simulink model "adcs_v11_log"  (Simulink 7.4)
settings: Solver=ode4  StartTime=0.0  StopTime=80000  FixedStep=s_SIM_STEP_SIZE  RelTol=1e-3
values from neighbouring files (symbols this model uses):
  A = ((T_SIDE + .29)*1e-3)^2    [constants_v13.m]    (also in constants_v15.m; constants_v15_Pow.m; constants_v15_Pow_ss_error.m; constants_v16_integral_kartavya.m)
  Ca_Solar_Drag = 1.4    [constants_v13.m]    (also in constants_v15.m = 0; constants_v15_Pow.m; constants_v15_Pow_ss_error.m; constants_v16_integral_kartavya.m)
  Cd = 2.2    [constants_v13.m]    (also in constants_v15.m = 0; constants_v15_Pow.m; constants_v15_Pow_ss_error.m; constants_v16_integral_kartavya.m)
  check_time = 60000    [constants_v13.m]    (also in constants_v15.m = 10000; constants_v15_Pow_ss_error.m = 10000; constants_v16_integral_kartavya.m = 10000; constants_v16_integral_light_sun_sgp_igrf_power_13Dec2011.m = 10000)
  equinox = datenum('21-Mar-2010 12:0:0')    [constants_v13.m]    (also in constants_v15.m; constants_v15_Pow.m = datenum('20-Mar-2015 12:0:0'); constants_v15_Pow_ss_error.m; constants_v16_integral_kartavya.m)
  err_SGP = 0    [constants_v16_integral_kartavya.m]    (also in constants_v16_integral_light_sun_sgp_igrf_power_13Dec2011.m)
  I_MAX = 0.5    [constants_v13.m]    (also in constants_v15.m; constants_v15_Pow.m; constants_v15_Pow_ss_error.m; constants_v16_integral_kartavya.m)
  I_TORQUER = 3.6 / 7.31    (= 0.492476060192)    [constants_v13.m]    (also in constants_v15.m = 0.272727272727; constants_v15_Pow.m; constants_v15_Pow_ss_error.m; constants_v16_integral_kartavya.m)
  Kd = 2* m_INERTIA / (s_numOrbits * T_ORBIT )    [constants_v13.m]    (also in constants_v15.m = m_INERTIA * (2 + delta)* zeta * w; constants_v15_Pow.m = m_INERTIA * (2 + delta)* zeta * w; constants_v15_Pow_ss_error.m = m_INERTIA * (2 + delta)* zeta * w; constants_v16_integral_kartavya.m = m_INERTIA * (2 + delta)* zeta * w)
  Kdetumb = K_det*eye(3)    [constants_v13.m]    (also in constants_v15.m; constants_v15_Pow.m; constants_v15_Pow_ss_error.m; constants_v16_integral_kartavya.m)
  Kp = m_INERTIA / (s_numOrbits * T_ORBIT * zeta)^2    [constants_v13.m]    (also in constants_v15.m = m_INERTIA * (w*w + 2*delta*zeta^2*w^2); constants_v15_Pow.m = m_INERTIA * (w*w + 2*delta*zeta^2*w^2); constants_v15_Pow_ss_error.m = m_INERTIA * (w*w + 2*delta*zeta^2*w^2); constants_v16_integral_kartavya.m = m_INERTIA * (w*w + 2*delta*zeta^2*w^2))
  m_INERTIA = [Ixx Ixy Ixz; Ixy Iyy Iyz; Ixz Iyz Izz]    [constants_v13.m]    (also in constants_v15.m; constants_v15_Pow.m = 1*[Ixx Ixy Ixz; Ixy Iyy Iyz; Ixz Iyz Izz]; constants_v15_Pow_ss_error.m = 1*[Ixx Ixy Ixz; Ixy Iyy Iyz; Ixz Iyz Izz]; constants_v16_integral_kartavya.m)
  mu = 6.673e-11*5.9742e24    (= 398658366000000)    [constants_v13.m]    (also in constants_v15.m; constants_v15_Pow.m; constants_v15_Pow_ss_error.m; constants_v16_integral_kartavya.m)
  N = 40    [constants_v13.m]    (also in constants_v15.m = 60; constants_v15_Pow.m; constants_v15_Pow_ss_error.m; constants_v16_integral_kartavya.m)
  P_momentum_flux_from_the_sun = 4.4e-6    (= 4.4e-06)    [constants_v13.m]    (also in constants_v15.m = 0; constants_v15_Pow.m; constants_v15_Pow_ss_error.m; constants_v16_integral_kartavya.m)
  q_BI0 = x_fromEnvModel(1:4)'    [OILS_script.m]    (also in OILS_script_OBC_preflight_bounce_back.m; OILS_script_extended.m; OILS_script_preflight_test.m; constants_v13.m = euler2qBI(roll0,pitch0,yaw0))
  s_AU = 159597870610    [constants_v16_integral_kartavya.m]    (also in constants_v16_integral_light_sun_sgp_igrf_power_13Dec2011.m; light_calc.m)
  s_DOY = sime(2)*30 - 30 + sime(3)    [constants_v16_integral_kartavya.m]    (also in constants_v16_integral_light_sun_sgp_igrf_power_13Dec2011.m; precalcs.m = doy(sime(3),sime(2),sime(3)))
  s_FRAME_SIZE = 2    [constants_v13.m]    (also in constants_v15.m; constants_v15_Pow.m; constants_v15_Pow_ss_error.m; constants_v16_integral_kartavya.m)
  s_m_MAX = 0.95    [constants_v13.m]    (also in constants_v15.m; constants_v15_Pow.m; constants_v15_Pow_ss_error.m; constants_v16_integral_kartavya.m)
  s_MAG_B = 2.5e-5    (= 2.5e-05)    [constants_v13.m]    (also in constants_v15.m; constants_v15_Pow.m; constants_v15_Pow_ss_error.m; constants_v16_integral_kartavya.m)
  s_MAGMETER_WEIGHT = .9    (= 0.9)    [constants_v13.m]    (also in constants_v15.m; constants_v15_Pow.m; constants_v15_Pow_ss_error.m; constants_v16_integral_kartavya.m)
  s_Rearth = 6378164    [constants_v16_integral_kartavya.m]    (also in constants_v16_integral_light_sun_sgp_igrf_power_13Dec2011.m; light_calc.m)
  s_Rsun = 695500000    [constants_v16_integral_kartavya.m]    (also in constants_v16_integral_light_sun_sgp_igrf_power_13Dec2011.m; light_calc.m)
  s_SEC = sime(4)*3600 + sime(5)*60 + sime(6)    [constants_v16_integral_kartavya.m]    (also in constants_v16_integral_light_sun_sgp_igrf_power_13Dec2011.m; precalcs.m)
  s_SIM_STEP_SIZE = 0.1    [constants_v13.m]    (also in constants_v15.m; constants_v15_Pow.m; constants_v15_Pow_ss_error.m; constants_v16_integral_kartavya.m)
  s_SS_ADC_gain = 5    [constants_v13.m]    (also in constants_v15.m = 3.3; constants_v15_Pow.m; constants_v15_Pow_ss_error.m; constants_v16_integral_kartavya.m)
  s_SS_ADC_res = 2^12 - 1    (= 4095)    [constants_v13.m]    (also in constants_v15.m = 1023; constants_v15_Pow.m; constants_v15_Pow_ss_error.m; constants_v16_integral_kartavya.m)
  s_SS_MAX_ANGLE = 85    [constants_v13.m]    (also in constants_v15.m = 55; constants_v15_Pow.m; constants_v15_Pow_ss_error.m; constants_v16_integral_kartavya.m)
  s_W_SAT = sqrt(mu/R_e^3)    [constants_v13.m]    (also in constants_v15.m; constants_v15_Pow.m; constants_v15_Pow_ss_error.m; constants_v16_integral_kartavya.m)
  s_x_MAGMETER_BIAS = 50e-9    (= 5e-08)    [constants_v13.m]    (also in constants_v15.m = 0; constants_v15_Pow.m; constants_v15_Pow_ss_error.m; constants_v16_integral_kartavya.m)
  s_YEAR = sime(1) + (sime(2)*30 - 30 + sime(3))/365    [constants_v16_integral_kartavya.m]    (also in constants_v16_integral_light_sun_sgp_igrf_power_13Dec2011.m; precalcs.m = decyear(sime); virtuallabexpt3mag.m = decyear(sime))
  side = 0.26    [constants_v13.m]    (also in constants_v15.m; constants_v15_Pow.m; constants_v15_Pow_ss_error.m; constants_v16_integral_kartavya.m)
  Snum = 6    [constants_v13.m]    (also in constants_v15.m; constants_v15_Pow.m; constants_v15_Pow_ss_error.m; constants_v16_integral_kartavya.m)
  stperut = 1.00273790935    [constants_v16_integral_kartavya.m]    (also in constants_v16_integral_light_sun_sgp_igrf_power_13Dec2011.m; precalcs.m; virtuallabexpt3mag.m)
  t_reset = 600    [constants_v16_integral_kartavya.m]    (also in constants_v16_integral_light_sun_sgp_igrf_power_13Dec2011.m; precalcs.m)
  TLE_epoch = datenum('18-Oct-2015 10:30:0')    [constants_v15.m]    (also in constants_v16_integral_kartavya.m = datenum('18-Oct-2010 10:30:0'); constants_v16_integral_light_sun_sgp_igrf_power_13Dec2011.m = datenum('18-Oct-2010 10:30:0'); precalcs.m)
  today = datenum('18-Oct-2010 10:30:0')    [constants_v13.m]    (also in constants_v15.m; constants_v15_Pow.m = datenum('18-Oct-2015 10:30:0'); constants_v15_Pow_ss_error.m; constants_v16_integral_kartavya.m)
  tol_w = 4e-3    (= 0.004)    [constants_v13.m]    (also in constants_v15.m; constants_v15_Pow.m; constants_v15_Pow_ss_error.m; constants_v16_integral_kartavya.m)
  Ts_display = 6    [constants_v13.m]    (also in constants_v15.m = 2; constants_v15_Pow.m; constants_v15_Pow_ss_error.m; constants_v16_integral_kartavya.m)
  v_COM_to_COP_b = [.2; 1.75; .2]*1e-2    [constants_v13.m]    (also in constants_v15.m = [.2; 1.75; .2]*0e-2; constants_v15_Pow.m; constants_v15_Pow_ss_error.m; constants_v16_integral_kartavya.m)
  v_S1 = [1 0 0]    [constants_v13.m]    (also in constants_v15.m; constants_v15_Pow.m; constants_v15_Pow_ss_error.m; constants_v16_integral_kartavya.m)
  v_S2 = [-1 0 0]    [constants_v13.m]    (also in constants_v15.m; constants_v15_Pow.m; constants_v15_Pow_ss_error.m; constants_v16_integral_kartavya.m)
  v_S3 = [0 1 0]    [constants_v13.m]    (also in constants_v15.m; constants_v15_Pow.m; constants_v15_Pow_ss_error.m; constants_v16_integral_kartavya.m)
  v_S4 = [0 -1 0]    [constants_v13.m]    (also in constants_v15.m; constants_v15_Pow.m; constants_v15_Pow_ss_error.m; constants_v16_integral_kartavya.m)
  v_S5 = [0 0 1]    [constants_v13.m]    (also in constants_v15.m; constants_v15_Pow.m; constants_v15_Pow_ss_error.m; constants_v16_integral_kartavya.m)
  v_S6 = [0 0 -1]    [constants_v13.m]    (also in constants_v15.m; constants_v15_Pow.m; constants_v15_Pow_ss_error.m; constants_v16_integral_kartavya.m)
  v_x_MOUNTING_THETA_ZYX_BODY_TORQUER = [1; 1; 1]* pi/180    [constants_v13.m]    (also in constants_v15.m; constants_v15_Pow.m; constants_v15_Pow_ss_error.m; constants_v16_integral_kartavya.m)
  W_EARTH_ROT = 2*pi/86400    (= 7.27220521664e-05)    [constants_v16_integral_kartavya.m]    (also in constants_v16_integral_light_sun_sgp_igrf_power_13Dec2011.m; precalcs.m; virtuallabexpt3mag.m)
  wx0 = x_fromEnvModel(5)    [OILS_script.m]    (also in OILS_script_OBC_preflight_bounce_back.m; OILS_script_extended.m; OILS_script_preflight_test.m; constants_v13.m = 0.0349065850399)
  wy0 = x_fromEnvModel(6)    [OILS_script.m]    (also in OILS_script_OBC_preflight_bounce_back.m; OILS_script_extended.m; OILS_script_preflight_test.m; constants_v13.m = 0.0174532925199)
  wz0 = x_fromEnvModel(7)    [OILS_script.m]    (also in OILS_script_OBC_preflight_bounce_back.m; OILS_script_extended.m; OILS_script_preflight_test.m; constants_v13.m = -0.0349065850399)
undefined symbols (not defined in the file or in its folder): Earth, s_omega_MAX, s_YEAR_ONLY, tol_pitch, tol_roll, tol_yaw, v_S10, v_S11, v_S12, v_S7, v_S8, v_S9, v_Si0, WGS84
libraries: commnoisgen2 x15, aerolibutil x7, aerolibtransform2 x5, dspsigops x5, powerlib_extras x3, aerolibgravity2 x2, aerolibatmos2 x1, dspmtrx3 x1, simulink x1
(part 2 of 3)

== system adcs_v11_log/Satellite Computations I Propagators/WMM/Subsystem ==
  Clock : Clock
      settings: Decimation=10
  m_DCM_ECI-ECEF2 : Stateflow chart
  today : Constant  Value=today  OutDataType=sfix(16)  OutScaling=2^0
  today1 : Constant  Value=equinox  OutDataType=sfix(16)  OutScaling=2^0
  today2 : Constant  Value=stperut  OutDataType=sfix(16)  OutScaling=2^0
  today3 : Constant  Value=W_EARTH_ROT  OutDataType=sfix(16)  OutScaling=2^0
  TEI : Outport
  wires:
  m_DCM_ECI-ECEF2/1(TEI) -> TEI/1
  Clock/1 -> m_DCM_ECI-ECEF2/5(t)
  today3/1 -> m_DCM_ECI-ECEF2/4(W_EARTH_ROT)
  today2/1 -> m_DCM_ECI-ECEF2/3(stperut)
  today1/1 -> m_DCM_ECI-ECEF2/2(equinox)
  today/1 -> m_DCM_ECI-ECEF2/1(today)

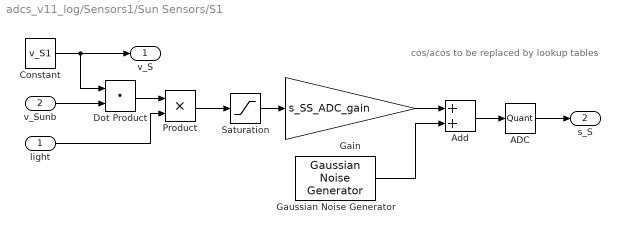
== system adcs_v11_log/Sensors1/Sun Sensors/S1 ==
  note: cos/acos to be replaced by lookup tables
  light : Inport  OutDataType=sfix(16)  OutScaling=2^0
  v_Sunb : Inport  Port=2  OutDataType=sfix(16)  OutScaling=2^0
  ADC : Quantizer  QuantizationInterval=1/s_SS_ADC_res
  Add : Sum  OutDataType=sfix(16)  OutScaling=2^-10
  Constant : Constant  Value=v_S1  OutDataType=sfix(16)  OutScaling=2^0
  Dot Product : DotProduct  OutDataType=sfix(16)  OutScaling=2^-10  InputSameDT=on  OutDataTypeStr=Inherit: Inherit via internal rule
  Gain : Gain  Gain=s_SS_ADC_gain  ParameterDataType=sfix(16)  ParameterScaling=2^0  OutDataType=sfix(16)  OutScaling=2^0
  Gaussian Noise Generator : commnoisgen2/Gaussian Noise Generator  SystemSampleTime=-1  m=0  d=s_x_SUNSENSOR  s=41  Ts=s_SIM_STEP_SIZE  frameBased=off  sampPerFrame=1  orient=off  outDataType=double
  Product : Product  OutDataType=fixdt(1, 16)  OutScaling=2^0  RndMeth=Zero
  Saturation : Saturate  UpperLimit=inf  LowerLimit=0  OutDataType=sfix(16)  OutScaling=2^0
  v_S : Outport  OutDataType=sfix(16)  OutScaling=2^0
  s_S : Outport  Port=2  OutDataType=sfix(16)  OutScaling=2^0
  wires:
  light/1 -> Product/2
  Product/1 -> Saturation/1
  Dot Product/1 -> Product/1
  v_Sunb/1 -> Dot Product/2
  Saturation/1 -> Gain/1
  Constant/1 -> v_S/1, Dot Product/1
  Gaussian Noise Generator/1 -> Add/2
  Gain/1 -> Add/1
  Add/1 -> ADC/1
  ADC/1 -> s_S/1

== system adcs_v11_log/Sensors1/Sun Sensors/S10 ==
  note: cos/acos to be replaced by lookup tables
  light : Inport  OutDataType=sfix(16)  OutScaling=2^0
  v_Sunb : Inport  Port=2  OutDataType=sfix(16)  OutScaling=2^0
  ADC : Quantizer  QuantizationInterval=1/s_SS_ADC_res
  Add : Sum  OutDataType=sfix(16)  OutScaling=2^-10
  Constant : Constant  Value=v_S10  OutDataType=sfix(16)  OutScaling=2^0
  Dot Product : DotProduct  OutDataType=sfix(16)  OutScaling=2^-10  InputSameDT=on  OutDataTypeStr=Inherit: Inherit via internal rule
  Gain : Gain  Gain=s_SS_ADC_gain  ParameterDataType=sfix(16)  ParameterScaling=2^0  OutDataType=sfix(16)  OutScaling=2^0
  Gaussian Noise Generator : commnoisgen2/Gaussian Noise Generator  SystemSampleTime=-1  m=0  d=s_x_SUNSENSOR  s=41  Ts=s_SIM_STEP_SIZE  frameBased=off  sampPerFrame=1  orient=off  outDataType=double
  Product : Product  OutDataType=fixdt(1, 16)  OutScaling=2^0  RndMeth=Zero
  Saturation : Saturate  UpperLimit=inf  LowerLimit=0  OutDataType=sfix(16)  OutScaling=2^0
  v_S : Outport  OutDataType=sfix(16)  OutScaling=2^0
  s_S : Outport  Port=2  OutDataType=sfix(16)  OutScaling=2^0
  wires:
  ADC/1 -> s_S/1
  Add/1 -> ADC/1
  Gain/1 -> Add/1
  Gaussian Noise Generator/1 -> Add/2
  Constant/1 -> Dot Product/1, v_S/1
  Saturation/1 -> Gain/1
  v_Sunb/1 -> Dot Product/2
  Dot Product/1 -> Product/1
  Product/1 -> Saturation/1
  light/1 -> Product/2

== system adcs_v11_log/Sensors1/Sun Sensors/S11 ==
  note: cos/acos to be replaced by lookup tables
  light : Inport  OutDataType=sfix(16)  OutScaling=2^0
  v_Sunb : Inport  Port=2  OutDataType=sfix(16)  OutScaling=2^0
  ADC : Quantizer  QuantizationInterval=1/s_SS_ADC_res
  Add : Sum  OutDataType=sfix(16)  OutScaling=2^-10
  Constant : Constant  Value=v_S11  OutDataType=sfix(16)  OutScaling=2^0
  Dot Product : DotProduct  OutDataType=sfix(16)  OutScaling=2^-10  InputSameDT=on  OutDataTypeStr=Inherit: Inherit via internal rule
  Gain : Gain  Gain=s_SS_ADC_gain  ParameterDataType=sfix(16)  ParameterScaling=2^0  OutDataType=sfix(16)  OutScaling=2^0
  Gaussian Noise Generator : commnoisgen2/Gaussian Noise Generator  SystemSampleTime=-1  m=0  d=s_x_SUNSENSOR  s=41  Ts=s_SIM_STEP_SIZE  frameBased=off  sampPerFrame=1  orient=off  outDataType=double
  Product : Product  OutDataType=fixdt(1, 16)  OutScaling=2^0  RndMeth=Zero
  Saturation : Saturate  UpperLimit=inf  LowerLimit=0  OutDataType=sfix(16)  OutScaling=2^0
  v_S : Outport  OutDataType=sfix(16)  OutScaling=2^0
  s_S : Outport  Port=2  OutDataType=sfix(16)  OutScaling=2^0
  wires:
  light/1 -> Product/2
  Product/1 -> Saturation/1
  Dot Product/1 -> Product/1
  v_Sunb/1 -> Dot Product/2
  Saturation/1 -> Gain/1
  Constant/1 -> v_S/1, Dot Product/1
  Gaussian Noise Generator/1 -> Add/2
  Gain/1 -> Add/1
  Add/1 -> ADC/1
  ADC/1 -> s_S/1

== system adcs_v11_log/Sensors1/Sun Sensors/S12 ==
  note: cos/acos to be replaced by lookup tables
  light : Inport  OutDataType=sfix(16)  OutScaling=2^0
  v_Sunb : Inport  Port=2  OutDataType=sfix(16)  OutScaling=2^0
  ADC : Quantizer  QuantizationInterval=1/s_SS_ADC_res
  Add : Sum  OutDataType=sfix(16)  OutScaling=2^-10
  Constant : Constant  Value=v_S12  OutDataType=sfix(16)  OutScaling=2^0
  Dot Product : DotProduct  OutDataType=sfix(16)  OutScaling=2^-10  InputSameDT=on  OutDataTypeStr=Inherit: Inherit via internal rule
  Gain : Gain  Gain=s_SS_ADC_gain  ParameterDataType=sfix(16)  ParameterScaling=2^0  OutDataType=sfix(16)  OutScaling=2^0
  Gaussian Noise Generator : commnoisgen2/Gaussian Noise Generator  SystemSampleTime=-1  m=0  d=s_x_SUNSENSOR  s=41  Ts=s_SIM_STEP_SIZE  frameBased=off  sampPerFrame=1  orient=off  outDataType=double
  Product : Product  OutDataType=fixdt(1, 16)  OutScaling=2^0  RndMeth=Zero
  Saturation : Saturate  UpperLimit=inf  LowerLimit=0  OutDataType=sfix(16)  OutScaling=2^0
  v_S : Outport  OutDataType=sfix(16)  OutScaling=2^0
  s_S : Outport  Port=2  OutDataType=sfix(16)  OutScaling=2^0
  wires:
  ADC/1 -> s_S/1
  Add/1 -> ADC/1
  Gain/1 -> Add/1
  Gaussian Noise Generator/1 -> Add/2
  Constant/1 -> Dot Product/1, v_S/1
  Saturation/1 -> Gain/1
  v_Sunb/1 -> Dot Product/2
  Dot Product/1 -> Product/1
  Product/1 -> Saturation/1
  light/1 -> Product/2

== system adcs_v11_log/Sensors1/Sun Sensors/S2 ==
  note: cos/acos to be replaced by lookup tables
  light : Inport  OutDataType=sfix(16)  OutScaling=2^0
  v_Sunb : Inport  Port=2  OutDataType=sfix(16)  OutScaling=2^0
  ADC : Quantizer  QuantizationInterval=1/s_SS_ADC_res
  Add : Sum  OutDataType=sfix(16)  OutScaling=2^-10
  Constant : Constant  Value=v_S2  OutDataType=sfix(16)  OutScaling=2^0
  Dot Product : DotProduct  OutDataType=sfix(16)  OutScaling=2^-10  InputSameDT=on  OutDataTypeStr=Inherit: Inherit via internal rule
  Gain : Gain  Gain=s_SS_ADC_gain  ParameterDataType=sfix(16)  ParameterScaling=2^0  OutDataType=sfix(16)  OutScaling=2^0
  Gaussian Noise Generator : commnoisgen2/Gaussian Noise Generator  SystemSampleTime=-1  m=0  d=s_x_SUNSENSOR  s=41  Ts=s_SIM_STEP_SIZE  frameBased=off  sampPerFrame=1  orient=off  outDataType=double
  Product : Product  OutDataType=fixdt(1, 16)  OutScaling=2^0  RndMeth=Zero
  Saturation : Saturate  UpperLimit=inf  LowerLimit=0  OutDataType=sfix(16)  OutScaling=2^0
  v_S : Outport  OutDataType=sfix(16)  OutScaling=2^0
  s_S : Outport  Port=2  OutDataType=sfix(16)  OutScaling=2^0
  wires:
  ADC/1 -> s_S/1
  Add/1 -> ADC/1
  Gain/1 -> Add/1
  Gaussian Noise Generator/1 -> Add/2
  Constant/1 -> Dot Product/1, v_S/1
  Saturation/1 -> Gain/1
  v_Sunb/1 -> Dot Product/2
  Dot Product/1 -> Product/1
  Product/1 -> Saturation/1
  light/1 -> Product/2

== system adcs_v11_log/Sensors1/Sun Sensors/S3 ==
  note: cos/acos to be replaced by lookup tables
  light : Inport  OutDataType=sfix(16)  OutScaling=2^0
  v_Sunb : Inport  Port=2  OutDataType=sfix(16)  OutScaling=2^0
  ADC : Quantizer  QuantizationInterval=1/s_SS_ADC_res
  Add : Sum  OutDataType=sfix(16)  OutScaling=2^-10
  Constant : Constant  Value=v_S3  OutDataType=sfix(16)  OutScaling=2^0
  Dot Product : DotProduct  OutDataType=sfix(16)  OutScaling=2^-10  InputSameDT=on  OutDataTypeStr=Inherit: Inherit via internal rule
  Gain : Gain  Gain=s_SS_ADC_gain  ParameterDataType=sfix(16)  ParameterScaling=2^0  OutDataType=sfix(16)  OutScaling=2^0
  Gaussian Noise Generator : commnoisgen2/Gaussian Noise Generator  SystemSampleTime=-1  m=0  d=s_x_SUNSENSOR  s=41  Ts=s_SIM_STEP_SIZE  frameBased=off  sampPerFrame=1  orient=off  outDataType=double
  Product : Product  OutDataType=fixdt(1, 16)  OutScaling=2^0  RndMeth=Zero
  Saturation : Saturate  UpperLimit=inf  LowerLimit=0  OutDataType=sfix(16)  OutScaling=2^0
  v_S : Outport  OutDataType=sfix(16)  OutScaling=2^0
  s_S : Outport  Port=2  OutDataType=sfix(16)  OutScaling=2^0
  wires:
  light/1 -> Product/2
  Product/1 -> Saturation/1
  Dot Product/1 -> Product/1
  v_Sunb/1 -> Dot Product/2
  Saturation/1 -> Gain/1
  Constant/1 -> v_S/1, Dot Product/1
  Gaussian Noise Generator/1 -> Add/2
  Gain/1 -> Add/1
  Add/1 -> ADC/1
  ADC/1 -> s_S/1

== system adcs_v11_log/Sensors1/Sun Sensors/S4 ==
  note: cos/acos to be replaced by lookup tables
  light : Inport  OutDataType=sfix(16)  OutScaling=2^0
  v_Sunb : Inport  Port=2  OutDataType=sfix(16)  OutScaling=2^0
  ADC : Quantizer  QuantizationInterval=1/s_SS_ADC_res
  Add : Sum  OutDataType=sfix(16)  OutScaling=2^-10
  Constant : Constant  Value=v_S4  OutDataType=sfix(16)  OutScaling=2^0
  Dot Product : DotProduct  OutDataType=sfix(16)  OutScaling=2^-10  InputSameDT=on  OutDataTypeStr=Inherit: Inherit via internal rule
  Gain : Gain  Gain=s_SS_ADC_gain  ParameterDataType=sfix(16)  ParameterScaling=2^0  OutDataType=sfix(16)  OutScaling=2^0
  Gaussian Noise Generator : commnoisgen2/Gaussian Noise Generator  SystemSampleTime=-1  m=0  d=s_x_SUNSENSOR  s=41  Ts=s_SIM_STEP_SIZE  frameBased=off  sampPerFrame=1  orient=off  outDataType=double
  Product : Product  OutDataType=fixdt(1, 16)  OutScaling=2^0  RndMeth=Zero
  Saturation : Saturate  UpperLimit=inf  LowerLimit=0  OutDataType=sfix(16)  OutScaling=2^0
  v_S : Outport  OutDataType=sfix(16)  OutScaling=2^0
  s_S : Outport  Port=2  OutDataType=sfix(16)  OutScaling=2^0
  wires:
  ADC/1 -> s_S/1
  Add/1 -> ADC/1
  Gain/1 -> Add/1
  Gaussian Noise Generator/1 -> Add/2
  Constant/1 -> Dot Product/1, v_S/1
  Saturation/1 -> Gain/1
  v_Sunb/1 -> Dot Product/2
  Dot Product/1 -> Product/1
  Product/1 -> Saturation/1
  light/1 -> Product/2

== system adcs_v11_log/Sensors1/Sun Sensors/S5 ==
  note: cos/acos to be replaced by lookup tables
  light : Inport  OutDataType=sfix(16)  OutScaling=2^0
  v_Sunb : Inport  Port=2  OutDataType=sfix(16)  OutScaling=2^0
  ADC : Quantizer  QuantizationInterval=1/s_SS_ADC_res
  Add : Sum  OutDataType=sfix(16)  OutScaling=2^-10
  Constant : Constant  Value=v_S5  OutDataType=sfix(16)  OutScaling=2^0
  Dot Product : DotProduct  OutDataType=sfix(16)  OutScaling=2^-10  InputSameDT=on  OutDataTypeStr=Inherit: Inherit via internal rule
  Gain : Gain  Gain=s_SS_ADC_gain  ParameterDataType=sfix(16)  ParameterScaling=2^0  OutDataType=sfix(16)  OutScaling=2^0
  Gaussian Noise Generator : commnoisgen2/Gaussian Noise Generator  SystemSampleTime=-1  m=0  d=s_x_SUNSENSOR  s=41  Ts=s_SIM_STEP_SIZE  frameBased=off  sampPerFrame=1  orient=off  outDataType=double
  Product : Product  OutDataType=fixdt(1, 16)  OutScaling=2^0  RndMeth=Zero
  Saturation : Saturate  UpperLimit=inf  LowerLimit=0  OutDataType=sfix(16)  OutScaling=2^0
  v_S : Outport  OutDataType=sfix(16)  OutScaling=2^0
  s_S : Outport  Port=2  OutDataType=sfix(16)  OutScaling=2^0
  wires:
  light/1 -> Product/2
  Product/1 -> Saturation/1
  Dot Product/1 -> Product/1
  v_Sunb/1 -> Dot Product/2
  Saturation/1 -> Gain/1
  Constant/1 -> v_S/1, Dot Product/1
  Gaussian Noise Generator/1 -> Add/2
  Gain/1 -> Add/1
  Add/1 -> ADC/1
  ADC/1 -> s_S/1

== system adcs_v11_log/Sensors1/Sun Sensors/S6 ==
  note: cos/acos to be replaced by lookup tables
  light : Inport  OutDataType=sfix(16)  OutScaling=2^0
  v_Sunb : Inport  Port=2  OutDataType=sfix(16)  OutScaling=2^0
  ADC : Quantizer  QuantizationInterval=1/s_SS_ADC_res
  Add : Sum  OutDataType=sfix(16)  OutScaling=2^-10
  Constant : Constant  Value=v_S6  OutDataType=sfix(16)  OutScaling=2^0
  Dot Product : DotProduct  OutDataType=sfix(16)  OutScaling=2^-10  InputSameDT=on  OutDataTypeStr=Inherit: Inherit via internal rule
  Gain : Gain  Gain=s_SS_ADC_gain  ParameterDataType=sfix(16)  ParameterScaling=2^0  OutDataType=sfix(16)  OutScaling=2^0
  Gaussian Noise Generator : commnoisgen2/Gaussian Noise Generator  SystemSampleTime=-1  m=0  d=s_x_SUNSENSOR  s=41  Ts=s_SIM_STEP_SIZE  frameBased=off  sampPerFrame=1  orient=off  outDataType=double
  Product : Product  OutDataType=fixdt(1, 16)  OutScaling=2^0  RndMeth=Zero
  Saturation : Saturate  UpperLimit=inf  LowerLimit=0  OutDataType=sfix(16)  OutScaling=2^0
  v_S : Outport  OutDataType=sfix(16)  OutScaling=2^0
  s_S : Outport  Port=2  OutDataType=sfix(16)  OutScaling=2^0
  wires:
  ADC/1 -> s_S/1
  Add/1 -> ADC/1
  Gain/1 -> Add/1
  Gaussian Noise Generator/1 -> Add/2
  Constant/1 -> Dot Product/1, v_S/1
  Saturation/1 -> Gain/1
  v_Sunb/1 -> Dot Product/2
  Dot Product/1 -> Product/1
  Product/1 -> Saturation/1
  light/1 -> Product/2

== system adcs_v11_log/Sensors1/Sun Sensors/S7 ==
  note: cos/acos to be replaced by lookup tables
  light : Inport  OutDataType=sfix(16)  OutScaling=2^0
  v_Sunb : Inport  Port=2  OutDataType=sfix(16)  OutScaling=2^0
  ADC : Quantizer  QuantizationInterval=1/s_SS_ADC_res
  Add : Sum  OutDataType=sfix(16)  OutScaling=2^-10
  Constant : Constant  Value=v_S7  OutDataType=sfix(16)  OutScaling=2^0
  Dot Product : DotProduct  OutDataType=sfix(16)  OutScaling=2^-10  InputSameDT=on  OutDataTypeStr=Inherit: Inherit via internal rule
  Gain : Gain  Gain=s_SS_ADC_gain  ParameterDataType=sfix(16)  ParameterScaling=2^0  OutDataType=sfix(16)  OutScaling=2^0
  Gaussian Noise Generator : commnoisgen2/Gaussian Noise Generator  SystemSampleTime=-1  m=0  d=s_x_SUNSENSOR  s=41  Ts=s_SIM_STEP_SIZE  frameBased=off  sampPerFrame=1  orient=off  outDataType=double
  Product : Product  OutDataType=fixdt(1, 16)  OutScaling=2^0  RndMeth=Zero
  Saturation : Saturate  UpperLimit=inf  LowerLimit=0  OutDataType=sfix(16)  OutScaling=2^0
  v_S : Outport  OutDataType=sfix(16)  OutScaling=2^0
  s_S : Outport  Port=2  OutDataType=sfix(16)  OutScaling=2^0
  wires:
  light/1 -> Product/2
  Product/1 -> Saturation/1
  Dot Product/1 -> Product/1
  v_Sunb/1 -> Dot Product/2
  Saturation/1 -> Gain/1
  Constant/1 -> v_S/1, Dot Product/1
  Gaussian Noise Generator/1 -> Add/2
  Gain/1 -> Add/1
  Add/1 -> ADC/1
  ADC/1 -> s_S/1

== system adcs_v11_log/Sensors1/Sun Sensors/S8 ==
  note: cos/acos to be replaced by lookup tables
  light : Inport  OutDataType=sfix(16)  OutScaling=2^0
  v_Sunb : Inport  Port=2  OutDataType=sfix(16)  OutScaling=2^0
  ADC : Quantizer  QuantizationInterval=1/s_SS_ADC_res
  Add : Sum  OutDataType=sfix(16)  OutScaling=2^-10
  Constant : Constant  Value=v_S8  OutDataType=sfix(16)  OutScaling=2^0
  Dot Product : DotProduct  OutDataType=sfix(16)  OutScaling=2^-10  InputSameDT=on  OutDataTypeStr=Inherit: Inherit via internal rule
  Gain : Gain  Gain=s_SS_ADC_gain  ParameterDataType=sfix(16)  ParameterScaling=2^0  OutDataType=sfix(16)  OutScaling=2^0
  Gaussian Noise Generator : commnoisgen2/Gaussian Noise Generator  SystemSampleTime=-1  m=0  d=s_x_SUNSENSOR  s=41  Ts=s_SIM_STEP_SIZE  frameBased=off  sampPerFrame=1  orient=off  outDataType=double
  Product : Product  OutDataType=fixdt(1, 16)  OutScaling=2^0  RndMeth=Zero
  Saturation : Saturate  UpperLimit=inf  LowerLimit=0  OutDataType=sfix(16)  OutScaling=2^0
  v_S : Outport  OutDataType=sfix(16)  OutScaling=2^0
  s_S : Outport  Port=2  OutDataType=sfix(16)  OutScaling=2^0
  wires:
  ADC/1 -> s_S/1
  Add/1 -> ADC/1
  Gain/1 -> Add/1
  Gaussian Noise Generator/1 -> Add/2
  Constant/1 -> Dot Product/1, v_S/1
  Saturation/1 -> Gain/1
  v_Sunb/1 -> Dot Product/2
  Dot Product/1 -> Product/1
  Product/1 -> Saturation/1
  light/1 -> Product/2

== system adcs_v11_log/Sensors1/Sun Sensors/S9 ==
  note: cos/acos to be replaced by lookup tables
  light : Inport  OutDataType=sfix(16)  OutScaling=2^0
  v_Sunb : Inport  Port=2  OutDataType=sfix(16)  OutScaling=2^0
  ADC : Quantizer  QuantizationInterval=1/s_SS_ADC_res
  Add : Sum  OutDataType=sfix(16)  OutScaling=2^-10
  Constant : Constant  Value=v_S9  OutDataType=sfix(16)  OutScaling=2^0
  Dot Product : DotProduct  OutDataType=sfix(16)  OutScaling=2^-10  InputSameDT=on  OutDataTypeStr=Inherit: Inherit via internal rule
  Gain : Gain  Gain=s_SS_ADC_gain  ParameterDataType=sfix(16)  ParameterScaling=2^0  OutDataType=sfix(16)  OutScaling=2^0
  Gaussian Noise Generator : commnoisgen2/Gaussian Noise Generator  SystemSampleTime=-1  m=0  d=s_x_SUNSENSOR  s=41  Ts=s_SIM_STEP_SIZE  frameBased=off  sampPerFrame=1  orient=off  outDataType=double
  Product : Product  OutDataType=fixdt(1, 16)  OutScaling=2^0  RndMeth=Zero
  Saturation : Saturate  UpperLimit=inf  LowerLimit=0  OutDataType=sfix(16)  OutScaling=2^0
  v_S : Outport  OutDataType=sfix(16)  OutScaling=2^0
  s_S : Outport  Port=2  OutDataType=sfix(16)  OutScaling=2^0
  wires:
  light/1 -> Product/2
  Product/1 -> Saturation/1
  Dot Product/1 -> Product/1
  v_Sunb/1 -> Dot Product/2
  Saturation/1 -> Gain/1
  Constant/1 -> v_S/1, Dot Product/1
  Gaussian Noise Generator/1 -> Add/2
  Gain/1 -> Add/1
  Add/1 -> ADC/1
  ADC/1 -> s_S/1

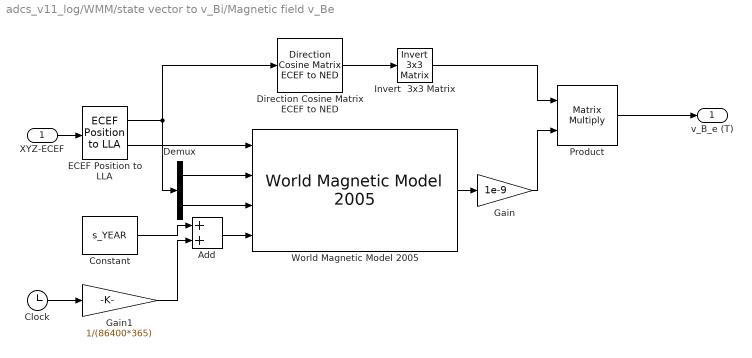
== system adcs_v11_log/WMM/state vector to v_Bi/Magnetic field v_Be ==
  XYZ-ECEF : Inport  OutDataType=sfix(16)  OutScaling=2^0
  Add : Sum  OutDataType=sfix(16)  OutScaling=2^-10
  Clock : Clock
      settings: Decimation=10
  Constant : Constant  Value=s_YEAR  OutDataType=sfix(16)  OutScaling=2^0
  Demux : Demux  Outputs=2
  Direction Cosine Matrix ECEF to NED : aerolibtransform2/Direction Cosine Matrix ECEF to NED  SystemSampleTime=-1
  ECEF Position to LLA : aerolibtransform2/ECEF Position to LLA  SystemSampleTime=-1  units=Metric (MKS)  ptype=Earth (WGS84)  F=1/298.257223563  R=6378137
  Gain : Gain  Gain=1e-9  ParameterDataType=sfix(16)  ParameterScaling=2^0  OutDataType=sfix(16)  OutScaling=2^0
  Gain1 : Gain  Gain=1/(86400*365)  ParameterDataType=sfix(16)  ParameterScaling=2^0  OutDataType=sfix(16)  OutScaling=2^0
  Invert  3x3 Matrix : aerolibutil/Invert  3x3 Matrix  SystemSampleTime=-1
  Product : Product  Multiplication=Matrix(*)  OutDataType=sfix(16)  OutScaling=2^0  RndMeth=Zero
  World Magnetic Model 2005 : aerolibgravity2/World Magnetic Model 2005  SystemSampleTime=-1  units=Metric (MKS)  time_in=on  month=January  day=1  year=2005  action=Error  h_out=off  dec_out=off  inc_out=off  ti_out=off
  "v_B_e (T) " : Outport  OutDataType=sfix(16)  OutScaling=2^0
  wires:
  Gain1/1 -> Add/2
  Clock/1 -> Gain1/1
  Add/1 -> World Magnetic Model 2005/4
  Constant/1 -> Add/1
  XYZ-ECEF/1 -> ECEF Position to LLA/1
  ECEF Position to LLA/1 -> Demux/1, Direction Cosine Matrix ECEF to NED/1
  ECEF Position to LLA/2 -> World Magnetic Model 2005/1
  Demux/1 -> World Magnetic Model 2005/2
  Demux/2 -> World Magnetic Model 2005/3
  Direction Cosine Matrix ECEF to NED/1 -> Invert  3x3 Matrix/1
  Invert  3x3 Matrix/1 -> Product/1
  Product/1 -> "v_B_e (T) "/1
  World Magnetic Model 2005/1 -> Gain/1
  Gain/1 -> Product/2

== system adcs_v11_log/WMM/state vector to v_Bi/Subsystem ==
  Clock : Clock
      settings: Decimation=10
  m_DCM_ECI-ECEF2 : Stateflow chart
  today : Constant  Value=today  OutDataType=sfix(16)  OutScaling=2^0
  today1 : Constant  Value=equinox  OutDataType=sfix(16)  OutScaling=2^0
  today2 : Constant  Value=stperut  OutDataType=sfix(16)  OutScaling=2^0
  today3 : Constant  Value=W_EARTH_ROT  OutDataType=sfix(16)  OutScaling=2^0
  TEI : Outport
  wires:
  m_DCM_ECI-ECEF2/1(TEI) -> TEI/1
  Clock/1 -> m_DCM_ECI-ECEF2/5(t)
  today3/1 -> m_DCM_ECI-ECEF2/4(W_EARTH_ROT)
  today2/1 -> m_DCM_ECI-ECEF2/3(stperut)
  today1/1 -> m_DCM_ECI-ECEF2/2(equinox)
  today/1 -> m_DCM_ECI-ECEF2/1(today)

== matlab function Torquer/Embedded MATLAB Function4 ==
  data: euler input double; DCM output double
function DCM  = f(euler)
% This block supports the Embedded MATLAB subset.
% See the help menu for details. 

roll = euler(1);
pitch = euler(2);
yaw = euler(3);

rot_x = [  1         0           0;...
             0         cos(roll)  sin(roll);...
             0        -sin(roll)  cos(roll)];
         
rot_y = [cos(pitch)   0       -sin(pitch);...
            0           1        0;...
           sin(pitch)   0        cos(pitch)];
       
rot_z = [ cos(yaw) sin(yaw) 0;...
           -sin(yaw) cos(yaw) 0;...
            0        0            1];
         
DCM  = rot_z *  rot_y *  rot_x;

== matlab function Embedded MATLAB Function ==
  data: x input double; u input double; xdot output double; m_INERTIA parameter double
function xdot = fcn(x, u, m_INERTIA)
% This block supports the Embedded MATLAB subset.
% See the help menu for details. 

q = x(1:4);
w = x(5:7);

W = ...
    [ 0 w(3) -w(2) w(1);
      -w(3) 0 w(1) w(2);
      w(2) -w(1) 0 w(3);
      -w(1) -w(2) -w(3) 0];
  
  qdot = 0.5 * W * q;
  wdot = inv(m_INERTIA)*( u - cross( w, m_INERTIA*w ) );
  
  xdot = [qdot; wdot];

== matlab function Subsystem/Sun Vector Propagator ==
  data: today input double; v_Sun_i output double; t input double
function v_Sun_i = fcn(today,t)
% This sun model block gives the sun vector in body frame.
% See the help menu for details. 

beta = 0;   %what is this? document this block.
time1 = today + t / 86400;
lambda = (2*pi*time1) / 365.256363;
epsilon = 23.5 * pi / 180;

sin_delta = cos(epsilon)*sin(beta) + sin(epsilon)*cos(beta)*sin(lambda);
delta = asin(sin_delta);

cos_alpha = cos(lambda) * cos(beta) / cos(delta);
alpha = acos(cos_alpha);
if (delta >= 0)
    alpha = alpha;
else
    alpha = (2*pi - 2*alpha) + alpha;
end

x = cos(delta)*cos(alpha);
y = cos(delta)*sin(alpha);
z = sin(delta);

v_Sun_i = [x; y; z];

== matlab function Subsystem/f: I->B ==
  data: x input double; v_B output double; v_I input double
function v_B = fcn(x, v_I)
% This block supports the Embedded MATLAB subset.
% See the help menu for details. 

q = x(1:4);

q0 = q(4); q1 = q(1); q2 = q(2); q3 = q(3);

TBI = [ q0^2 + q1^2 - q2^2 - q3^2,         2*q0*q3 + 2*q1*q2,         2*q1*q3 - 2*q0*q2;
           2*q1*q2 - 2*q0*q3, q0^2 - q1^2 + q2^2 - q3^2,         2*q0*q1 + 2*q2*q3;
           2*q0*q2 + 2*q1*q3,         2*q2*q3 - 2*q0*q1, q0^2 - q1^2 - q2^2 + q3^2];

v_B =  TBI*v_I;
v_B = v_B/sqrt(dot(v_B,v_B));

== matlab function WMM/L_Inertial ==
  data: x input double; v_B output double; v_I input double
function v_B = fcn(x, v_I)
% This block supports the Embedded MATLAB subset.
% See the help menu for details. 

q = x(1:4);

q0 = q(4); q1 = q(1); q2 = q(2); q3 = q(3);

TBI = [ q0^2 + q1^2 - q2^2 - q3^2,         2*q0*q3 + 2*q1*q2,         2*q1*q3 - 2*q0*q2;
           2*q1*q2 - 2*q0*q3, q0^2 - q1^2 + q2^2 - q3^2,         2*q0*q1 + 2*q2*q3;
           2*q0*q2 + 2*q1*q3,         2*q2*q3 - 2*q0*q1, q0^2 - q1^2 - q2^2 + q3^2];

v_B =  TBI*v_I;

== matlab function q -> w/Subsystem6/Embedded MATLAB Function ==
  data: a input double; y output double; b input double
function y = fcn(a,b)
%#eml

y = a+b;
if y>1
    y=1;
end

== matlab function q-normalise ==
  data: x input double; xN output double
function xN  = fcn(x)
% This block gives DCM for converting from ECI to ORBIT frames
% inputs: state vector in ECI
% output: DCM

q = x(1:4);
q = q/sqrt(dot(q,q));
xN = [q; x(5:7)];

== matlab function External Torques/Subsystem/Solar_drag ==
  data: v_Sun_b input double; solar_drag output double; Ca_Solar_Drag parameter double; P_momentum_flux_from_the_sun parameter double; light input double; side parameter double
function solar_drag = fcn(v_Sun_b,Ca_Solar_Drag,P_momentum_flux_from_the_sun,light, side)
% This block supports the Embedded MATLAB subset.
% See the help menu for details. 

% dot product of area vector and sun vector
if (norm(v_Sun_b) == 0)
    u = [1;0;0];
else
    u = v_Sun_b / norm(v_Sun_b);
end

y = 0 ;
a = side;
a = a*a; %Area of satellite
b =  zeros(3,6);
b(:,1) = a*[1;0;0];
b(:,2) = a*[0;1;0];
b(:,3) = a*[0;0;1];
b(:,4) = a*[-1;0;0];
b(:,5) = a*[0;-1;0];
b(:,6) = a*[0;0;-1];

x = 0;
for i=1:6
     x = dot(b(:,i),u);
    if(x>0)
            y = y+x;
    end
end
Ap = y;

solar_drag = -Ap * Ca_Solar_Drag * P_momentum_flux_from_the_sun * u * light;

== matlab function External Torques/L_Inertial ==
  data: x input double; tau output double; v_Si input double; mu parameter double; m_INERTIA parameter double
function tau = fcn(x, v_Si, mu, m_INERTIA)
% This block supports the Embedded MATLAB subset.
% See the help menu for details. 

q = x(1:4);

q0 = q(4); q1 = q(1); q2 = q(2); q3 = q(3);

TBI = [ q0^2 + q1^2 - q2^2 - q3^2,         2*q0*q3 + 2*q1*q2,         2*q1*q3 - 2*q0*q2;
           2*q1*q2 - 2*q0*q3, q0^2 - q1^2 + q2^2 - q3^2,         2*q0*q1 + 2*q2*q3;
           2*q0*q2 + 2*q1*q3,         2*q2*q3 - 2*q0*q1, q0^2 - q1^2 - q2^2 + q3^2];

r_I = v_Si(1:3);
r_B =  TBI*r_I;

R = sqrt(dot(r_B, r_B));
tau = 3*mu * cross( r_B, m_INERTIA*r_B) / R^5;

== matlab function Control Law/q->w ==
  data: B output double; B_l input double; B_k input double; dB output double; s_FRAME_SIZE parameter double
function [B, dB] = fcn(B_l, B_k, s_FRAME_SIZE)
% This block supports the Embedded MATLAB subset.
% See the help menu for details. 

dB = (B_l - B_k)/s_FRAME_SIZE;
B = (B_l + B_k)/2;

== matlab function QuEST ==
  data: v_Bb_m input double; m_SUN input double; q_BO_est output double; v_Bo_c input double; v_So_c input double; s_SS_ADC_gain parameter double; Snum parameter double; light_est output double; s_MAGMETER_WEIGHT parameter double; s_SS_MAX_ANGLE parameter double; v_Sun1 output double
function [q_BO_est, light_est, v_Sun1] = QuEST(v_Bb_m,m_SUN,v_Bo_c,v_So_c, s_SS_ADC_gain, Snum, s_MAGMETER_WEIGHT, s_SS_MAX_ANGLE)

    % Help
    % q_triad = Estimated quaternion
    % b1,b2 = the 2 measurement vectors in body frames
    % r1,r2 = the 2 measurement vectors in reference frames (orbit/inertial; orbit used)
    % b1 is the measurement with very high accurace as compared to b2
    % I am not sure how r1 and r2 will be determined
    % a1 and a2 are Relative weights of b1 and b2


%%%%% calculate v_Sb_m from m_SUN %%%%
t_S = ones(1,Snum)*cos(s_SS_MAX_ANGLE *pi/180);
m_SUN(4,:) = 1.0*(m_SUN(5,:)>t_S);     % set flags from measured voltages

values = m_SUN(5,:);

n_SS = 0;
for i=1:Snum
    if values(i) < 0.5*s_SS_ADC_gain
        n_SS = n_SS + 1;
    end
end

if (n_SS == Snum) 
    light = 0;
else
    light = 1;
end

light_est = light;
%v_Sun1 = [1;0;0];

if (light == 1)    
    
    ssvectors = zeros(3); ssvalues = zeros(3,1); ssflags = zeros(3,1);
     % flags = m_SUN(4,:)';
    for i=1:3
        [~, index] = sort(m_SUN(5,:));  % sort values in ascending order
        z = index(Snum);
        ssvectors(i,1:3) = m_SUN(1:3,z)';
        ssflags(i) = m_SUN(4,z);
        ssvalues(i) = m_SUN(5,z);
        m_SUN(5,z) = -100 ;
        for j= 1:Snum
            if( norm(ssvectors(i,1:3)+m_SUN(1:3,j)') == 0 )
                m_SUN(5,j) = -100;
            end
        end
    end
    
    % v_Sun1 = inv(ssvectors)*ssvalues;
    v_Sun1 = ssvectors\ssvalues;
    v_Sun1 = v_Sun1/sqrt(dot(v_Sun1, v_Sun1));
    v_Sb_m = v_Sun1/sqrt(dot(v_Sun1, v_Sun1));
    
    %%%% start TRIAD %%%%

    b1 = v_Bb_m;
    b2 = v_Sb_m;
    r1 = v_Bo_c;
    r2 = v_So_c;

    a1 = s_MAGMETER_WEIGHT;
    a2 = 1-a1;

    %b3
    b3 = cross(b1,b2);
    b3 = b3/norm(b3) ;
    %r3
    r3 = cross(r1,r2);
    r3 = r3/norm(r3) ;

    %mu
    mu = ( 1 + dot(b3,r3) ) * ( a1*dot(b1,r1) + a2*dot(b2,r2) ) ;
    mu =  mu + dot( cross(b3,r3) , ( a1*cross(b1,r1) + a2*cross(b2,r2) ) ) ;

    %nu
    nu = dot( ( b3 + r3 ) , ( a1*cross(b1,r1) + a2*cross(b2,r2) )  ) ;

    %rho
    rho = sqrt( mu*mu + nu*nu );

    %q
    if( mu > 0)
        k_q_triad = (1/( 2*sqrt( rho*(rho+mu)*( 1 + dot(b3,r3) ) ) ) );
        v_q_triad = ( rho + mu )*( cross(b3,r3) ) + nu*(b3 + r3) ;
        s_q_triad = ( rho + mu )* ( 1 + dot(b3,r3) ) ;
        q_triad = [v_q_triad ; s_q_triad];
        q_triad = k_q_triad * q_triad ;
    else
        k_q_triad = (1/( 2*sqrt( rho*(rho-mu)*( 1 + dot(b3,r3) ) ) ) );
        v_q_triad = ( nu )*( cross(b3,r3) ) + ( rho - mu )*(b3 + r3) ;
        s_q_triad = ( nu )* ( 1 + dot(b3,r3) ) ;
        q_triad = [v_q_triad ; s_q_triad];
        q_triad = k_q_triad * q_triad ;    
    end

    q_triad = q_triad / sqrt(dot(q_triad,q_triad)) ;
    q_BO_est = q_triad;
else
    v_Sun1 = [1 ; 0 ; 0];
    q_BO_est = [0;0;0;1];
    flag_sum = 0;
end
end

== matlab function Satellite Computations I Propagators/m_TOI_NEW1 ==
  data: v_I input double; ECI input double; v_O output double
function v_O  = fcn(v_I, ECI)
% This block gives DCM for converting from ECI to ORBIT frames
% inputs: state vector in ECI
% output: DCM

r = ECI(1:3);   % position vector in ECI
v = ECI(4:6);   % velocity vector in ECI

oy = cross(v,r);    % orbit frame x...
oy = oy/sqrt(dot(oy,oy));

oz = -r/sqrt(dot(r,r));

ox = cross(oy,oz);
ox = ox/sqrt(dot(ox,ox));

TOI = [ox oy oz]';

v_O = TOI*v_I;

== matlab function Control Law/Nominal ==
  data: eu output double; w_temp output double; light input double; w input double; m_N output double; v_B input double; Kp parameter double; Kd parameter double; s_MAG_B parameter double; q input double; s_W_SAT parameter double; s_omega_MAX parameter double
function [eu,w_temp,m_N] = fcn(light, w, v_B, Kp, Kd, s_MAG_B, q, s_W_SAT,s_omega_MAX)
% This block supports the Embedded MATLAB subset.
% See the help menu for details. 

Bnorm = sqrt(dot(v_B, v_B));
w_temp = w;

% %%Saturation
% if( w(1) > s_omega_MAX)
%     w_temp(1) = s_omega_MAX;
% elseif( w(1) < -s_omega_MAX)
%     w_temp(1) = -s_omega_MAX;
% end
% 
% if( w(2) > s_omega_MAX)
%     w_temp(2) = s_omega_MAX;
% elseif( w(2) < -s_omega_MAX)
%     w_temp(2) = -s_omega_MAX;
% end
% 
% if( w(3) > s_omega_MAX)
%     w_temp(3) = s_omega_MAX;
% elseif( w(3) < -s_omega_MAX)
%     w_temp(3) = -s_omega_MAX;    
% end
% %% Saturation Ends

q = q/sqrt(dot(q,q));

qv = q(1:3);    % e*sin(t/2)
qs = q(4);      %   cos(t/2)

eu = 2*qv*qs;     % 2*e*sin(t/2)*cos(t/2) = e*sin(t)
% q_BO = q;
% eu = [atan2( 2*( q_BO(4)*q_BO(1)-q_BO(2)*q_BO(3) ),( 1 - 2*( q_BO(1)^2 + q_BO(2)^2 ) )  ) ;
%        asin( 2*( q_BO(4)*q_BO(2)+q_BO(3)*q_BO(1)) );
%       atan2( 2*( q_BO(4)*q_BO(3)-q_BO(1)*q_BO(2) ),( 1 - 2*( q_BO(2)^2 + q_BO(3)^2 ) )  ) ];
         
mp = Kp * eu / Bnorm^2;
md = Kd * w_temp  / Bnorm^2;

m_N = cross( mp+md, v_B ) * light;

== matlab function WMM/state vector to v_Bi/Subsystem/m_DCM_ECI-ECEF2 ==
  data: TEI output double; today input double; equinox input double; stperut input double; W_EARTH_ROT input double; t input double
function TEI = fcn(today,equinox, stperut,W_EARTH_ROT,t)
% This block gives DCM for converting from ECI to ECEF frames
% inputs: today's date, equinox, sidereal time per unit time, angular velocity of earth's rotation, simulation time
% output: DCM

% 23hr 56m 4.09s per day

ut_sec = (today - equinox)*24*60*60 + t; % universal time in sec
st_sec = stperut*ut_sec;    % sidereal time in sec

phi = st_sec*W_EARTH_ROT;            % sidereal time in rad

TEI = [ cos(phi) sin(phi) 0;
       -sin(phi) cos(phi) 0;
        0        0        1];

== matlab function Satellite Computations I Propagators/Subsystem/Embedded MATLAB Function ==
  data: today input double; v_Sun_i output double; t input double
function v_Sun_i = fcn(today,t)
% This sun model block gives the sun vector in body frame.
% See the help menu for details. 

beta = 0;
time1 = today + t / 86400;
lambda = (2*pi*time1) / 365.256363;
epsilon = 23.5 * pi / 180;

sin_delta = cos(epsilon)*sin(beta) + sin(epsilon)*cos(beta)*sin(lambda);
delta = asin(sin_delta);

cos_alpha = cos(lambda) * cos(beta) / cos(delta);
alpha = acos(cos_alpha);
if (delta >= 0)
    alpha = alpha;
else
    alpha = (2*pi - 2*alpha) + alpha;
end

x = cos(delta)*cos(alpha);
y = cos(delta)*sin(alpha);
z = sin(delta);

v_Sun_i = [x; y; z];

== matlab function External Torques/Aerodynamic Torque/aero torque ==
  data: rho input double; v_B input double; u_aero output double; side parameter double; Cd parameter double; v_COM_to_COP_b parameter double
function u_aero = fcn(rho, v_B,side, Cd, v_COM_to_COP_b)

% x = 1;
% z = x*1;
% y = z*u;

% This block supports an embeddable subset of the MATLAB language.
% See the help menu for details. 
% dot product of area vector and velocity vector

vnorm = sqrt(dot(v_B,v_B));
v_unit = v_B / vnorm;

y = 0 ;
a = side;
a = a*a; %Area of satellite
b =  zeros(3,6);
b(:,1) = a*[1;0;0];
b(:,2) = a*[0;1;0];
b(:,3) = a*[0;0;1];
b(:,4) = a*[-1;0;0];
b(:,5) = a*[0;-1;0];
b(:,6) = a*[0;0;-1];

for i=1:6
     x = dot(b(:,i),v_unit);
    if(x>0)
            y = y+x;
    end
end
Ap = y; % total exposed area

F_aero = -0.5 * Cd * rho * Ap * vnorm^2 * v_unit;

u_aero = cross(v_COM_to_COP_b, F_aero);

== matlab function External Torques/Aerodynamic Torque/Subsystem/m_DCM_ECI-ECEF2 ==
  data: TEI output double; today input double; equinox input double; stperut input double; W_EARTH_ROT input double; t input double
function TEI = fcn(today,equinox, stperut,W_EARTH_ROT,t)
% This block gives DCM for converting from ECI to ECEF frames
% inputs: today's date, equinox, sidereal time per unit time, angular velocity of earth's rotation, simulation time
% output: DCM

% 23hr 56m 4.09s per day

ut_sec = (today - equinox)*24*60*60 + t; % universal time in sec
st_sec = stperut*ut_sec;    % sidereal time in sec

phi = st_sec*W_EARTH_ROT;            % sidereal time in rad

TEI = [ cos(phi) sin(phi) 0;
       -sin(phi) cos(phi) 0;
        0        0        1];

== matlab function Satellite Computations I Propagators/WMM/Subsystem/m_DCM_ECI-ECEF2 ==
  data: TEI output double; today input double; equinox input double; stperut input double; W_EARTH_ROT input double; t input double
function TEI = fcn(today,equinox, stperut,W_EARTH_ROT,t)
% This block gives DCM for converting from ECI to ECEF frames
% inputs: today's date, equinox, sidereal time per unit time, angular velocity of earth's rotation, simulation time
% output: DCM

% 23hr 56m 4.09s per day

ut_sec = (today - equinox)*24*60*60 + t; % universal time in sec
st_sec = stperut*ut_sec;    % sidereal time in sec

phi = st_sec*W_EARTH_ROT;            % sidereal time in rad

TEI = [ cos(phi) sin(phi) 0;
       -sin(phi) cos(phi) 0;
        0        0        1];

== matlab function External Torques/Aerodynamic Torque/rho(6) ==
  data: v_rho input double; rho output double
function rho = fcn(v_rho)
% This block supports the Embedded MATLAB subset.
% See the help menu for details. 

rho = v_rho(6);

end

== matlab function External Torques/Aerodynamic Torque/v_I to v_B ==
  data: v_I input double; x input double; v_B output double
function v_B = fcn(v_I,x)
% This block supports the Embedded MATLAB subset.
% See the help menu for details. 

q = x(1:4);

q0 = q(4); q1 = q(1); q2 = q(2); q3 = q(3);

TBI = [ q0^2 + q1^2 - q2^2 - q3^2,         2*q0*q3 + 2*q1*q2,         2*q1*q3 - 2*q0*q2;
           2*q1*q2 - 2*q0*q3, q0^2 - q1^2 + q2^2 - q3^2,         2*q0*q1 + 2*q2*q3;
           2*q0*q2 + 2*q1*q3,         2*q2*q3 - 2*q0*q1, q0^2 - q1^2 - q2^2 + q3^2];

v_B =  TBI*v_I;

== matlab function Eclipse model/Eclipse Model ==
  data: s_AU input double; flag output double; s_Rearth input double; s_Rsun input double; v_S_i input double; v_Sun_i input double; alpha output double; beta output double; parameter_umbra output double; parameter_penumbra output double
function [flag, alpha, beta, parameter_umbra, parameter_penumbra] = fcn(s_AU, s_Rearth, s_Rsun, v_S_i, v_Sun_i)
% This block supports the Embedded MATLAB subset.
% See the help menu for details. 

%159597870610 m = 1 AU
%695500000 m = Sun radius

v_pos_S_i = v_S_i(1:3);

umbra = s_AU*s_Rearth / (s_Rsun - s_Rearth);
penumbra = s_AU*s_Rearth / (s_Rsun + s_Rearth);

alpha = asin(s_Rearth / umbra);
beta = asin(s_Rearth / penumbra);

angle_sat = acos(dot(v_pos_S_i, v_Sun_i) / norm(v_pos_S_i));

parameter_umbra = acos((dot((v_pos_S_i + umbra*v_Sun_i), v_Sun_i)) / norm(v_pos_S_i + umbra*v_Sun_i));
parameter_penumbra = acos((dot((v_pos_S_i - penumbra*v_Sun_i), -v_Sun_i)) / norm(v_pos_S_i - penumbra*v_Sun_i));

flag = 1;

if ((angle_sat >= pi/2 + alpha) && (parameter_umbra <= alpha))
    flag = 0;
elseif ((angle_sat >= pi/2 + beta) && (parameter_umbra > alpha) && (parameter_penumbra <= beta))
        flag = 0.5;
end

== matlab function Sensors1/Sun Sensors/Embedded MATLAB Function ==
  data: v_S1 input double; m_SUN output double; s_S1 input double; v_S2 input double; s_S2 input double; v_S3 input double; s_S3 input double; v_S4 input double; s_S4 input double; v_S5 input double; s_S5 input double; v_S6 input double; s_S6 input double; v_S7 input double; s_S7 input double; v_S8 input double; s_S8 input double; v_S9 input double; s_S9 input double; v_S10 input double; s_S10 input double; v_S11 input double; s_S11 input double; v_S12 input double; s_S12 input double; Snum parameter double; s_SS_MAX_ANGLE parameter double; values output double
function [m_SUN, values] = fcn(v_S1, s_S1, v_S2, s_S2, v_S3, s_S3, v_S4, s_S4, v_S5, s_S5, v_S6, s_S6, v_S7, s_S7, v_S8, s_S8, v_S9, s_S9, v_S10, s_S10, v_S11, s_S11, v_S12, s_S12, Snum, s_SS_MAX_ANGLE)

a = cos(s_SS_MAX_ANGLE *pi/180);
t_S = ones(1,12)*a;

m_SUNtot = [v_S1 v_S2 v_S3 v_S4 v_S5 v_S6 v_S7 v_S8 v_S9 v_S10 v_S11 v_S12; % SS vectors
               0    0    0    0    0    0    0    0    0     0     0     0; % flags
            s_S1 s_S2 s_S3 s_S4 s_S5 s_S6 s_S7 s_S8 s_S9 s_S10 s_S11 s_S12];% values
        
m_SUNtot(4,:) = 1.0*(m_SUNtot(5,:)>t_S);

m_SUN = m_SUNtot(:, 1:Snum);
values = m_SUN(5,:)';

% [sorted, index] = sort(values);
% 
% 
% z = index(Snum-2:Snum);
% sunflags = [m_SUN(4,z(1)) m_SUN(4,z(2)) m_SUN(4,z(3))];
% sunvectors = [m_SUN(1:3,z(1)) m_SUN(1:3,z(2)) m_SUN(1:3,z(3))]';
% sunvalues = [m_SUN(5,z(1)); m_SUN(5,z(2)); m_SUN(5,z(3))];
% 
% vSun = inv(sunvectors)*sunvalues;
% 
% if (sqrt(dot(vSun,vSun)) > .1)
%     vSun = vSun/sqrt(dot(vSun,vSun));
% else
%     vSun = [0;0;0];
% end
%

== matlab function Control Law/Detumbling ==
  data: v_B input double; Bdot input double; Kdetumb parameter double; m_D output double; s_MAG_B parameter double
function m_D = fcn(v_B, Bdot, Kdetumb, s_MAG_B)
% This block supports the Embedded MATLAB subset.
% See the help menu for details. 

Bnorm = sqrt(dot(v_B, v_B));
m_D = -Kdetumb * Bdot * (s_MAG_B / Bnorm);

== matlab function Control Law/Switching Algorithm/gate pulse ==
  data: w input double; q input double; tol_w parameter double; N output double; tol_roll parameter double; tol_pitch parameter double; tol_yaw parameter double; t input double; check_time parameter double; light_flag input double; w_ctrl input double; time1 output double; time2 input double
function [N,time1] = fcn( w, q, tol_w, tol_roll, tol_pitch, tol_yaw, t,check_time, light_flag, w_ctrl,time2)

modw = sqrt(dot(w, w));
switch_condition = (abs(q(4)) > .6) && (modw < tol_w) && (light_flag ==1) && (w_ctrl == 1);

if (t<100)
    time1=0;
else
    time1=time2;
end

if ( switch_condition )
    N = 1; time1 =t;
elseif (time1==0)
    N=0; time1=0;
elseif (t > (check_time+time1))
    N = 0;
else
    N=1;
end

== matlab function Satellite Computations I Propagators/m_TOI_NEW ==
  data: ECI input double; v_O output double; v_I input double
function v_O  = fcn(ECI, v_I)
% This block gives DCM for converting from ECI to ORBIT frames
% inputs: state vector in ECI
% output: DCM

r = ECI(1:3);   % position vector in ECI
v = ECI(4:6);   % velocity vector in ECI

oy = cross(v,r);    % orbit frame x...
oy = oy/sqrt(dot(oy,oy));

oz = -r/sqrt(dot(r,r));

ox = cross(oy,oz);
ox = ox/sqrt(dot(ox,ox));

TOI = [ox oy oz]';

v_O = TOI*v_I;
